simulink model "codeModel"  (Simulink 6.6)
settings: Solver=ode45  StartTime=0.0  StopTime=10.0  RelTol=1e-3
undefined symbols (not defined in the file or in its folder): Active_Flags, Output
libraries: simulink x1
settings Model: Creator=Administrator  LastModifiedBy=Administrator

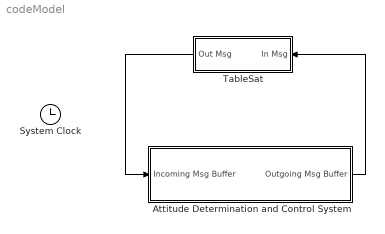
== system codeModel ==
  Attitude Determination and Control System : Subsystem
  System Clock : Clock
      settings: Decimation=10
  TableSat : Subsystem  Orientation=left
  wires:
  TableSat/1(Out Msg) -> Attitude Determination and Control System/1(Incoming Msg Buffer)
  Attitude Determination and Control System/1(Outgoing Msg Buffer) -> TableSat/1(In Msg)

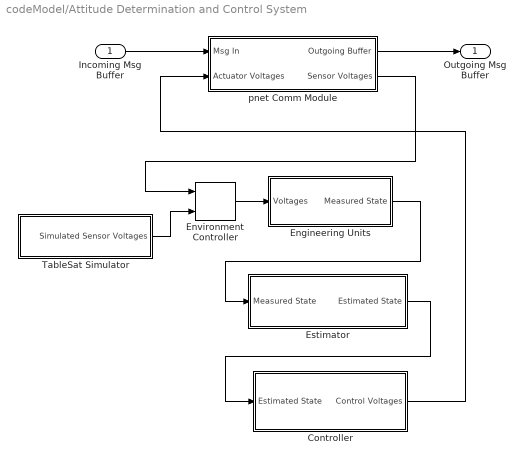
== system codeModel/Attitude Determination and Control System ==
  Incoming Msg Buffer : Inport
  Controller : Subsystem
  Engineering Units : Subsystem
  Environment Controller : simulink/Signal Routing/Environment Controller  SystemSampleTime=-1
  Estimator : Subsystem
  TableSat Simulator : Subsystem
  pnet Comm Module : Subsystem
  Outgoing Msg Buffer : Outport
  wires:
  TableSat Simulator/1(Simulated Sensor Voltages) -> Environment Controller/2
  Environment Controller/1 -> Engineering Units/1(Voltages)
  Engineering Units/1(Measured State) -> Estimator/1(Measured State)
  Estimator/1(Estimated State) -> Controller/1(Estimated State)
  Incoming Msg Buffer/1 -> pnet Comm Module/1(Msg In)
  pnet Comm Module/2(Sensor Voltages) -> Environment Controller/1
  pnet Comm Module/1(Outgoing Buffer) -> Outgoing Msg Buffer/1
  Controller/1(Control Voltages) -> pnet Comm Module/2(Actuator Voltages)

== system codeModel/TableSat ==
  In Msg : Inport
  Out Msg : Outport
  wires:
  In Msg/1 -> Out Msg/1

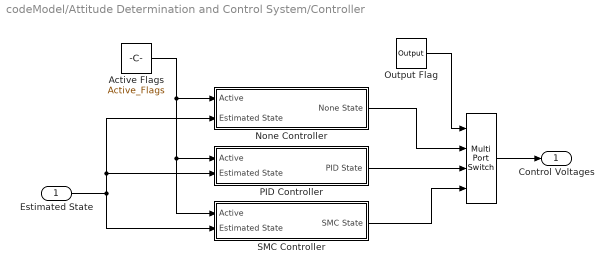
== system codeModel/Attitude Determination and Control System/Controller ==
  Estimated State : Inport
  " " : MultiPortSwitch  Inputs=3
  Active Flags : Constant  Value=Active_Flags
  None Controller : Subsystem
  Output Flag : Constant  Value=Output
  PID Controller : Subsystem
  SMC Controller : Subsystem
  Control Voltages : Outport
  wires:
  Estimated State/1 -> PID Controller/2(Estimated State), None Controller/2(Estimated State), SMC Controller/2(Estimated State)
  Active Flags/1 -> None Controller/1(Active), PID Controller/1(Active), SMC Controller/1(Active)
  Output Flag/1 -> " "/1
  " "/1 -> Control Voltages/1
  None Controller/1(None State) -> " "/2
  PID Controller/1(PID State) -> " "/3
  SMC Controller/1(SMC State) -> " "/4

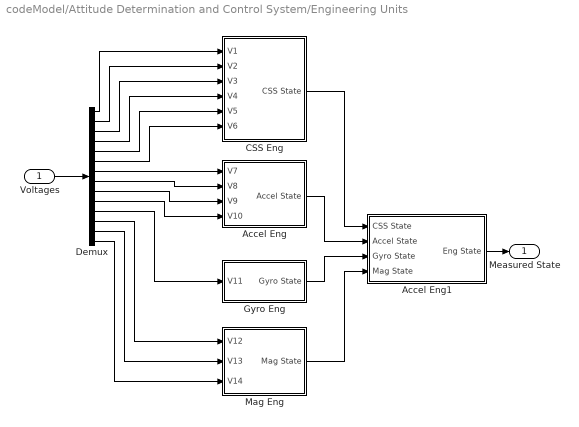
== system codeModel/Attitude Determination and Control System/Engineering Units ==
  Voltages : Inport
  Accel Eng : Subsystem
  Accel Eng1 : Subsystem
  CSS Eng : Subsystem
  Demux : Demux  Outputs=14
  Gyro Eng : Subsystem
  Mag Eng : Subsystem
  Measured State : Outport
  wires:
  Voltages/1 -> Demux/1
  Demux/1 -> CSS Eng/1(V1)
  Demux/2 -> CSS Eng/2(V2)
  Demux/3 -> CSS Eng/3(V3)
  Demux/4 -> CSS Eng/4(V4)
  Demux/5 -> CSS Eng/5(V5)
  Demux/6 -> CSS Eng/6(V6)
  Demux/7 -> Accel Eng/1(V7)
  Demux/8 -> Accel Eng/2(V8)
  Demux/9 -> Accel Eng/3(V9)
  Demux/10 -> Accel Eng/4(V10)
  Demux/11 -> Gyro Eng/1(V11)
  Demux/12 -> Mag Eng/1(V12)
  Demux/13 -> Mag Eng/2(V13)
  Demux/14 -> Mag Eng/3(V14)
  Accel Eng1/1(Eng State) -> Measured State/1
  CSS Eng/1(CSS State) -> Accel Eng1/1(CSS State)
  Accel Eng/1(Accel State) -> Accel Eng1/2(Accel State)
  Gyro Eng/1(Gyro State) -> Accel Eng1/3(Gyro State)
  Mag Eng/1(Mag State) -> Accel Eng1/4(Mag State)

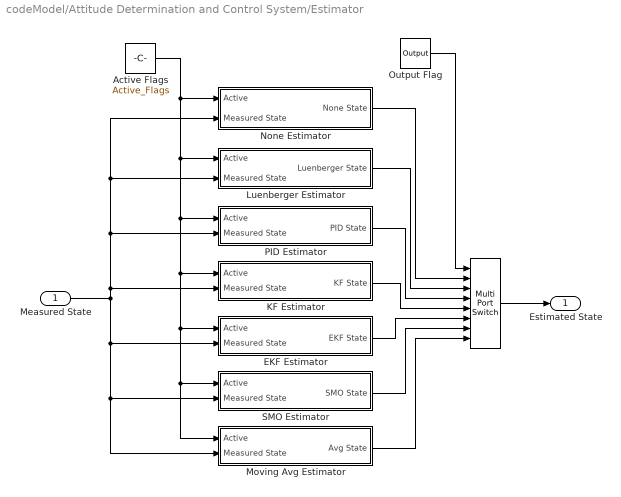
== system codeModel/Attitude Determination and Control System/Estimator ==
  Measured State : Inport
  " " : MultiPortSwitch  Inputs=7
  Active Flags : Constant  Value=Active_Flags
  EKF Estimator : Subsystem
  KF Estimator : Subsystem
  Luenberger Estimator : Subsystem
  Moving Avg Estimator : Subsystem
  None Estimator : Subsystem
  Output Flag : Constant  Value=Output
  PID Estimator : Subsystem
  SMO Estimator : Subsystem
  Estimated State : Outport
  wires:
  Measured State/1 -> None Estimator/2(Measured State), Luenberger Estimator/2(Measured State), PID Estimator/2(Measured State), KF Estimator/2(Measured State), EKF Estimator/2(Measured State), SMO Estimator/2(Measured State), Moving Avg Estimator/2(Measured State)
  Active Flags/1 -> None Estimator/1(Active), Luenberger Estimator/1(Active), PID Estimator/1(Active), KF Estimator/1(Active), EKF Estimator/1(Active), SMO Estimator/1(Active), Moving Avg Estimator/1(Active)
  Output Flag/1 -> " "/1
  None Estimator/1(None State) -> " "/2
  Luenberger Estimator/1(Luenberger State) -> " "/3
  PID Estimator/1(PID State) -> " "/4
  KF Estimator/1(KF State) -> " "/5
  EKF Estimator/1(EKF State) -> " "/6
  SMO Estimator/1(SMO State) -> " "/7
  Moving Avg Estimator/1(Avg State) -> " "/8
  " "/1 -> Estimated State/1

== system codeModel/Attitude Determination and Control System/TableSat Simulator ==
  RPM : Constant  Value=3
  Simulated Sensor Voltages : Outport

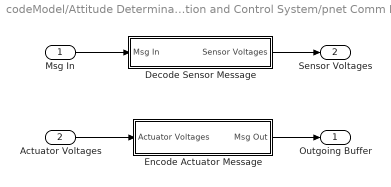
== system codeModel/Attitude Determination and Control System/pnet Comm Module ==
  Msg In : Inport
  Actuator Voltages : Inport  Port=2
  "Decode Sensor Message " : Subsystem
  Encode Actuator Message : Subsystem
  Outgoing Buffer : Outport
  Sensor Voltages : Outport  Port=2
  wires:
  "Decode Sensor Message "/1(Sensor Voltages) -> Sensor Voltages/1
  Msg In/1 -> "Decode Sensor Message "/1(Msg In)
  Actuator Voltages/1 -> Encode Actuator Message/1(Actuator Voltages)
  Encode Actuator Message/1(Msg Out) -> Outgoing Buffer/1

== system codeModel/Attitude Determination and Control System/Controller/None Controller ==
  Active : Inport
  Estimated State : Inport  Port=2
  None State : Outport
  wires:
  Estimated State/1 -> None State/1

== system codeModel/Attitude Determination and Control System/Controller/PID Controller ==
  Active : Inport
  Estimated State : Inport  Port=2
  PID State : Outport
  wires:
  Estimated State/1 -> PID State/1

== system codeModel/Attitude Determination and Control System/Controller/SMC Controller ==
  Active : Inport
  Estimated State : Inport  Port=2
  SMC State : Outport
  wires:
  Estimated State/1 -> SMC State/1

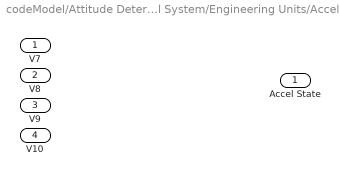
== system codeModel/Attitude Determination and Control System/Engineering Units/Accel Eng ==
  V7 : Inport
  V8 : Inport  Port=2
  V9 : Inport  Port=3
  V10 : Inport  Port=4
  Accel State : Outport

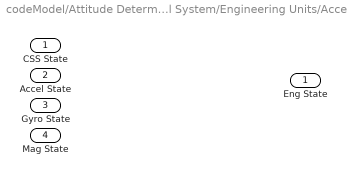
== system codeModel/Attitude Determination and Control System/Engineering Units/Accel Eng1 ==
  CSS State : Inport
  Accel State : Inport  Port=2
  Gyro State : Inport  Port=3
  Mag State : Inport  Port=4
  Eng State : Outport

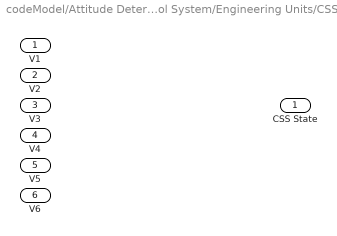
== system codeModel/Attitude Determination and Control System/Engineering Units/CSS Eng ==
  V1 : Inport
  V2 : Inport  Port=2
  V3 : Inport  Port=3
  V4 : Inport  Port=4
  V5 : Inport  Port=5
  V6 : Inport  Port=6
  CSS State : Outport

== system codeModel/Attitude Determination and Control System/Engineering Units/Gyro Eng ==
  V11 : Inport
  Gyro State : Outport

== system codeModel/Attitude Determination and Control System/Engineering Units/Mag Eng ==
  V12 : Inport
  V13 : Inport  Port=2
  V14 : Inport  Port=3
  Mag State : Outport

== system codeModel/Attitude Determination and Control System/Estimator/EKF Estimator ==
  Active : Inport
  Measured State : Inport  Port=2
  EKF State : Outport
  wires:
  Measured State/1 -> EKF State/1

== system codeModel/Attitude Determination and Control System/Estimator/KF Estimator ==
  Active : Inport
  Measured State : Inport  Port=2
  KF State : Outport
  wires:
  Measured State/1 -> KF State/1

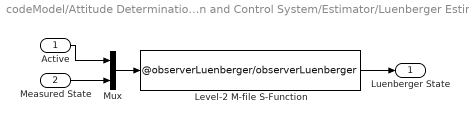
== system codeModel/Attitude Determination and Control System/Estimator/Luenberger Estimator ==
  Active : Inport
  Measured State : Inport  Port=2
  Level-2 M-file S-Function : M-S-Function  FunctionName=@observerLuenberger/observerLuenberger
  Mux : Mux  Inputs=2
  Luenberger State : Outport
  wires:
  Level-2 M-file S-Function/1 -> Luenberger State/1
  Active/1 -> Mux/1
  Measured State/1 -> Mux/2
  Mux/1 -> Level-2 M-file S-Function/1

== system codeModel/Attitude Determination and Control System/Estimator/Moving Avg Estimator ==
  Active : Inport
  Measured State : Inport  Port=2
  Avg State : Outport
  wires:
  Measured State/1 -> Avg State/1

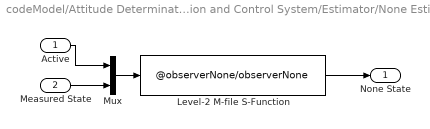
== system codeModel/Attitude Determination and Control System/Estimator/None Estimator ==
  Active : Inport
  Measured State : Inport  Port=2
  Level-2 M-file S-Function : M-S-Function  FunctionName=@observerNone/observerNone
  Mux : Mux  Inputs=2
  None State : Outport
  wires:
  Active/1 -> Mux/1
  Measured State/1 -> Mux/2
  Mux/1 -> Level-2 M-file S-Function/1
  Level-2 M-file S-Function/1 -> None State/1

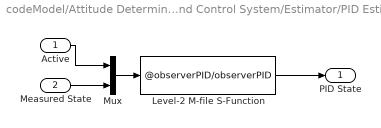
== system codeModel/Attitude Determination and Control System/Estimator/PID Estimator ==
  Active : Inport
  Measured State : Inport  Port=2
  Level-2 M-file S-Function : M-S-Function  FunctionName=@observerPID/observerPID
  Mux : Mux  Inputs=2
  PID State : Outport
  wires:
  Active/1 -> Mux/1
  Measured State/1 -> Mux/2
  Mux/1 -> Level-2 M-file S-Function/1
  Level-2 M-file S-Function/1 -> PID State/1

== system codeModel/Attitude Determination and Control System/Estimator/SMO Estimator ==
  Active : Inport
  Measured State : Inport  Port=2
  SMO State : Outport
  wires:
  Measured State/1 -> SMO State/1

== system codeModel/Attitude Determination and Control System/pnet Comm Module/Decode Sensor Message  ==
  Msg In : Inport
  Sensor Voltages : Outport

== system codeModel/Attitude Determination and Control System/pnet Comm Module/Encode Actuator Message ==
  Actuator Voltages : Inport
  Msg Out : Outport
